simulink model "soes_ethercat_slave_32bytes"  (R2018b)
settings: Solver=FixedStepDiscrete  StartTime=0.0  StopTime=100  FixedStep=0.05  RelTol=1e-3  EnableMultiTasking=on
undefined symbols (not defined in the file): Green, led0
libraries: embdlinuxlib x1
settings Model: FPTRunName=Active  ExtModeTrigDuration=2  Creator=ihout  LastModifiedBy=ihout
settings SolverCC: PositivePriorityOrder=on
settings DataIOCC: LimitDataPoints=on  SaveFormat=Array
settings OptimizationCC: ExpressionDepthLimit=2147483647  LifeSpan=Inf  MaxStackSize=64  SimCompilerOptimization=on
settings DebuggingCC: UnderspecifiedInitializationDetection=Classic  MergeDetectMultiDrivingBlocksExec=none  FcnCallInpInsideContextMsg=warning  AllowSymbolicDim=off  StateNameClashWarn=warning  SFUnexpectedBacktrackingDiag=warning  SFNoUnconditionalDefaultTransitionDiag=warning  SFExecutionAtInitializationDiag=none
settings HardwareCC: ProdBitPerPointer=32  ProdBitPerSizeT=32  ProdBitPerPtrDiffT=32  ProdLargestAtomicInteger=Long  ProdLargestAtomicFloat=Double  ProdWordSize=32  ProdHWDeviceType=ARM Compatible->ARM Cortex  UseEmbeddedCoderFeatures=off  UseSimulinkCoderFeatures=off
settings ModelReferenceCC: PropagateSignalLabelsOutOfModel=off
settings SFSimCC: SimUseLocalCustomCode=off
settings RTWCC: SystemTargetFile=ert.tlc  HardwareBoard=Raspberry Pi  TemplateMakefile=ert_default_tmf  GenerateReport=on  RTWVerbose=off  RTWUseLocalCustomCode=off  Toolchain=GNU GCC Raspberry Pi  BuildConfiguration=Faster Runs  LaunchReport=on
settings CodeAppCC: ForceParamTrailComments=on  OperatorAnnotations=on  StateflowObjectComments=on  MATLABSourceComments=on
settings ERTTargetCC: MultiwordLength=2048  ERTCustomFileBanners=off  SupportContinuousTime=on  SupportNonInlinedSFcns=on  RemoveResetFunc=off  SupportVariableSizeSignals=on  ModelStepFunctionPrototypeControlCompliant=off
settings ConfigComp: CovMetricSettings=dw  CovHtmlReporting=on  CovSaveCumulativeToWorkspaceVar=on  CovSaveSingleToWorkspaceVar=on  CovExternalEMLEnable=off  CovSFcnEnable=off

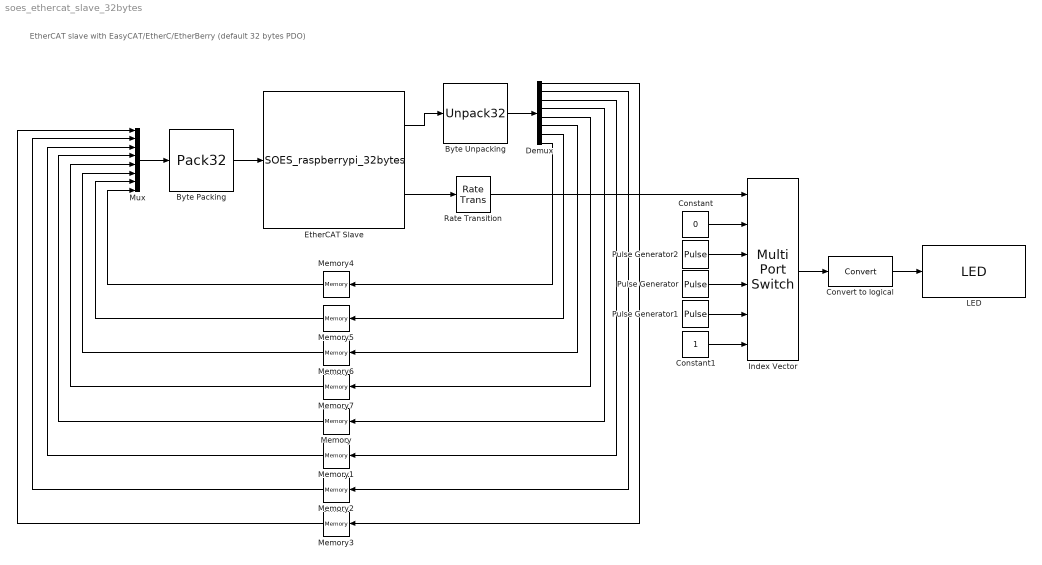
== system soes_ethercat_slave_32bytes ==
  note: EtherCAT slave with EasyCAT/EtherC/EtherBerry (default 32 bytes PDO)
  Byte Packing : S-Function  InitFcn=try, set_param(gcb,'FunctionName','Pack32'), end  FunctionName=Pack32  SFunctionModules=Pack32_wrapper  SFunctionDeploymentMode=off  EnableBusSupport=off  mask(S-Function Builder){}
      mask help: Simulink:masks:SFunctionBuilder_MD
      mask init:
      | val = [[.9  0.75 0.75 1 1 .9 .9 1]',[1 1 0.75 0.75 .9 .9 1 .9]'];try , sys = get_param(gcb,'SfunBuilderFcnName');if isempty(sys), sys = get_param(gcb,'FunctionName'); end,catch, sys = get_param(gcb,'FunctionName'); end
      settings: CopyFcn=set_param(gcbh,'LinkStatus','none')  PreSaveFcn=try, set_param(gcb,'FunctionName','Pack32'), end  OpenFcn=sfunctionwizard(gcbh)
      mask Display: plot(val(:,1),val(:,2)),disp(sys), port_label('input',1,'u'), port_label('output',1,'y')
  Byte Unpacking : S-Function  InitFcn=try, set_param(gcb,'FunctionName','Unpack32'), end  FunctionName=Unpack32  SFunctionModules=Unpack32_wrapper  SFunctionDeploymentMode=off  EnableBusSupport=off  mask(S-Function Builder){}
      mask help: Simulink:masks:SFunctionBuilder_MD
      mask init: same as soes_ethercat_slave_32bytes/Byte Packing
      settings: CopyFcn=set_param(gcbh,'LinkStatus','none')  PreSaveFcn=try, set_param(gcb,'FunctionName','Unpack32'), end  OpenFcn=sfunctionwizard(gcbh)
      mask Display: plot(val(:,1),val(:,2)),disp(sys), port_label('input',1,'u'), port_label('output',1,'y')
  Constant : Constant  Value=0  SampleTime=0.1
  Constant1 : Constant  SampleTime=0.1
  Convert to logical : DataTypeConversion
  Demux : Demux  Outputs=8
  EtherCAT Slave : S-Function  InitFcn=try, set_param(gcb,'FunctionName','SOES_raspberrypi_32bytes'), end  FunctionName=SOES_raspberrypi_32bytes  SFunctionModules=SOES_raspberrypi_32bytes_wrapper slave_objectlist  SFunctionDeploymentMode=off  EnableBusSupport=off  mask(S-Function Builder){}
      mask init: same as soes_ethercat_slave_32bytes/Byte Packing
      settings: CopyFcn=set_param(gcbh,'LinkStatus','none')  PreSaveFcn=try, set_param(gcb,'FunctionName','SOES_raspberrypi_32bytes'), end  OpenFcn=sfunctionwizard(gcbh)
      mask Display: plot(val(:,1),val(:,2)),disp(sys), port_label('input',1,'TxPdo'), port_label('output',1,'RxPdo'), port_label('output',2,'Status')
  Index Vector : MultiPortSwitch  DataPortOrder=Specify indices  Inputs=5  DataPortIndices={1,2,3,4,8}
  LED : embdlinuxlib/LED  board=Pi 3 Model B  led=led0 (Green)  blockPlatform=Raspberry Pi
      settings: SourceProductBaseCode=SC_BEAGLEBONE_BLUE,RASPPI
  Memory{,1..7} (8 alike) : Memory
  Mux : Mux  Inputs=8
  Pulse Generator : DiscretePulseGenerator  Period=10  PulseWidth=5  SampleTime=0.1
  Pulse Generator1 : DiscretePulseGenerator  Period=6  PulseWidth=3  SampleTime=0.1
  Pulse Generator2 : DiscretePulseGenerator  Period=20  PulseWidth=10  SampleTime=0.1
  Rate Transition : RateTransition  OutPortSampleTime=0.1
  wires:
  Byte Packing/1 -> EtherCAT Slave/1
  EtherCAT Slave/1 -> Byte Unpacking/1
  Mux/1 -> Byte Packing/1
  Memory/1 -> Mux/4
  Demux/4 -> Memory/1
  Memory1/1 -> Mux/3
  Demux/3 -> Memory1/1
  Demux/2 -> Memory2/1
  Demux/1 -> Memory3/1
  Memory2/1 -> Mux/2
  Memory3/1 -> Mux/1
  EtherCAT Slave/2 -> Rate Transition/1
  Index Vector/1 -> Convert to logical/1
  Convert to logical/1 -> LED/1
  Constant/1 -> Index Vector/2
  Pulse Generator1/1 -> Index Vector/5
  Pulse Generator/1 -> Index Vector/4
  Pulse Generator2/1 -> Index Vector/3
  Constant1/1 -> Index Vector/6
  Rate Transition/1 -> Index Vector/1
  Demux/5 -> Memory7/1
  Demux/6 -> Memory6/1
  Demux/7 -> Memory5/1
  Demux/8 -> Memory4/1
  Memory7/1 -> Mux/5
  Memory6/1 -> Mux/6
  Memory5/1 -> Mux/7
  Memory4/1 -> Mux/8
  Byte Unpacking/1 -> Demux/1
